simulink model "scheme1"  (R2024a)
settings: Solver=VariableStepAuto  StartTime=0.0  StopTime=10  RelTol=1e-3
libraries: simulink x1
settings Model: Creator=ventus  LastModifiedBy=ventus

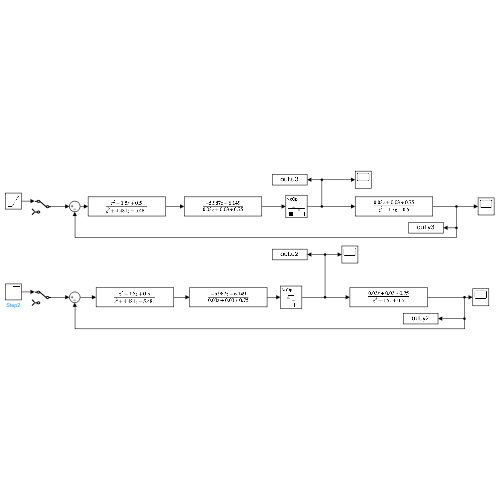
[thumbnail: Simulink's stored preview of the top-level diagram]
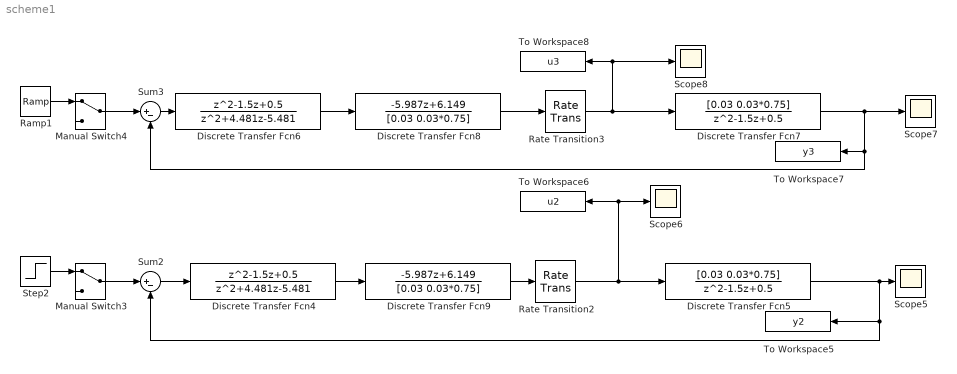
== system scheme1 ==
  Discrete Transfer Fcn4 : DiscreteTransferFcn  Numerator=[1 -1.5 0.5]  Denominator=[1 4.481 -5.481]
  Discrete Transfer Fcn5 : DiscreteTransferFcn  Numerator=[0.03 0.03*0.75]  Denominator=[1 -1.5 0.5]
  Discrete Transfer Fcn6 : DiscreteTransferFcn  Numerator=[1 -1.5 0.5]  Denominator=[1 4.481 -5.481]
  Discrete Transfer Fcn7 : DiscreteTransferFcn  Numerator=[0.03 0.03*0.75]  Denominator=[1 -1.5 0.5]
  Discrete Transfer Fcn8 : DiscreteTransferFcn  Numerator=[-5.987 6.149]  Denominator=[0.03 0.03*0.75]
  Discrete Transfer Fcn9 : DiscreteTransferFcn  Numerator=[-5.987 6.149]  Denominator=[0.03 0.03*0.75]
  Manual Switch3 : ManualSwitch
  Manual Switch4 : ManualSwitch
  Ramp1 : simulink/Sources/Ramp  slope=1  start=0  InitialOutput=0
  Rate Transition2 : RateTransition  OutPortSampleTime=0.1
  Rate Transition3 : RateTransition  OutPortSampleTime=0.1
  Scope{5..8} (4 alike) : Scope
  Step2 : Step  SampleTime=0
  Sum2 : Sum  Inputs=|+-
  Sum3 : Sum  Inputs=|+-
  To Workspace5 : ToWorkspace  VariableName=y2  SaveFormat=Timeseries  SampleTime=-1
  To Workspace6 : ToWorkspace  VariableName=u2  SaveFormat=Timeseries  SampleTime=-1
  To Workspace7 : ToWorkspace  VariableName=y3  SaveFormat=Timeseries  SampleTime=-1
  To Workspace8 : ToWorkspace  VariableName=u3  SaveFormat=Timeseries  SampleTime=-1
  wires:
  Discrete Transfer Fcn9/1 -> Rate Transition2/1
  Manual Switch4/1 -> Sum3/1
  Rate Transition3/1 -> Scope8/1, To Workspace8/1, Discrete Transfer Fcn7/1
  Discrete Transfer Fcn4/1 -> Discrete Transfer Fcn9/1
  Discrete Transfer Fcn7/1 -> To Workspace7/1, Sum3/2, Scope7/1
  Sum3/1 -> Discrete Transfer Fcn6/1
  Sum2/1 -> Discrete Transfer Fcn4/1
  Discrete Transfer Fcn6/1 -> Discrete Transfer Fcn8/1
  Step2/1 -> Manual Switch3/1
  Discrete Transfer Fcn5/1 -> To Workspace5/1, Sum2/2, Scope5/1
  Ramp1/1 -> Manual Switch4/1
  Discrete Transfer Fcn8/1 -> Rate Transition3/1
  Rate Transition2/1 -> Discrete Transfer Fcn5/1, To Workspace6/1, Scope6/1
  Manual Switch3/1 -> Sum2/1
